simulink model "TRAMI_TM_CNT"  (R2018b)
settings: Solver=ode8  StartTime=0  StopTime=end_time  FixedStep=sampling_time  RelTol=1e-3
PreLoadFcn:
  | TRAMI_TM_CNT_PreLoad;
libraries: simulink x1
settings Model: Creator=nishimura  LastModifiedBy=E00026
settings DataIOCC: LimitDataPoints=on  SaveFormat=Array  SaveOutput=off  InspectSignalLogs=on  SaveTime=off
settings OptimizationCC: BlockReduction=off  BooleanDataType=off  LifeSpan=inf
settings DebuggingCC: SaveWithParameterizedLinksMsg=none  UnderspecifiedInitializationDetection=Classic  MergeDetectMultiDrivingBlocksExec=none  SignalResolutionControl=TryResolveAllWithWarning  ParameterPrecisionLossMsg=none  StrictBusMsg=ErrorOnBusTreatedAsVector  SFUnexpectedBacktrackingDiag=warning  SFNoUnconditionalDefaultTransitionDiag=warning  SFExecutionAtInitializationDiag=none
settings HardwareCC: ProdBitPerPointer=32  ProdBitPerSizeT=32  ProdBitPerPtrDiffT=32  ProdLargestAtomicFloat=None  ProdIntDivRoundTo=Undefined  ProdEndianess=Unspecified  ProdWordSize=32  ProdHWDeviceType=32-bit Generic  TargetUnknown=on
settings ModelReferenceCC: PropagateSignalLabelsOutOfModel=off
settings SFSimCC: SimUseLocalCustomCode=off
settings RTWCC: RTWUseLocalCustomCode=off
settings CodeAppCC: StateflowObjectComments=on
settings GRTTargetCC: TargetLangStandard=C89/C90 (ANSI)  GeneratePreprocessorConditionals=Disable all
settings ConfigComp: CovMetricSettings=dw  CovHtmlReporting=on  CovSaveCumulativeToWorkspaceVar=on  CovSaveSingleToWorkspaceVar=on  CovExternalEMLEnable=off  CovSFcnEnable=off

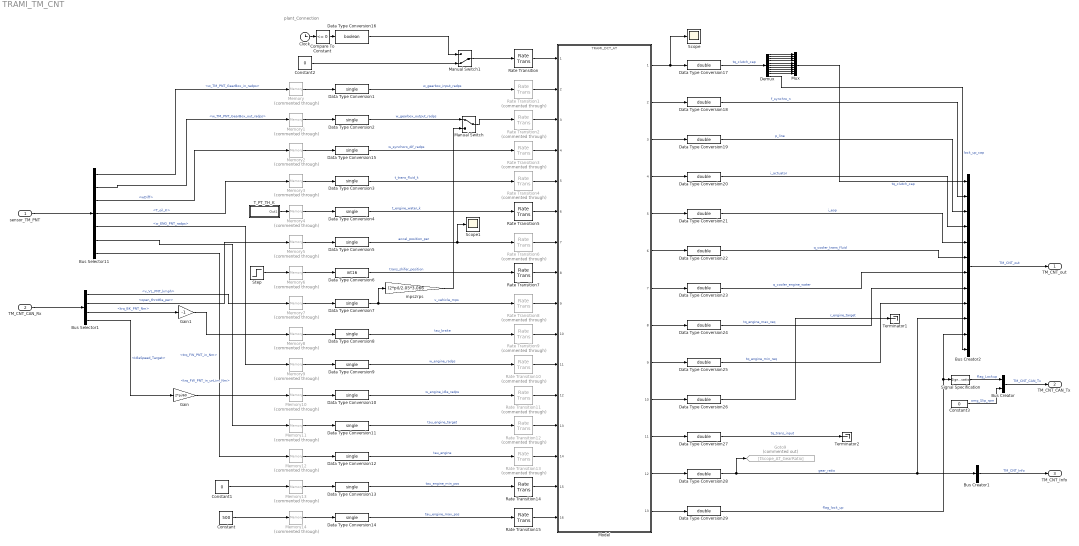
== system TRAMI_TM_CNT ==
  note: plant_Connection
  sensor_TM_PNT : Inport  OutDataTypeStr=Bus: sensor_TM_PNT_TRAMI  SampleTime=0.01
      settings: AttributesFormatString=|
      | <SampleTime = %<SampleTime>>
      | <%<OutDataTypeStr>>
  TM_CNT_CAN_Rx : Inport  Port=2  OutDataTypeStr=Bus: TM_CNT_CAN_Rx  SampleTime=0.01
      settings: AttributesFormatString=|
      | <SampleTime = %<SampleTime>>
      | <%<OutDataTypeStr>>
  Bus Creator : BusCreator  Inputs=2
  Bus Creator1 : BusCreator  Inputs=1
  Bus Creator2 : BusCreator  Inputs=12
  Bus Selector1 : BusSelector  OutputSignals=v_VL_PNT_kmph,open_throttle_per,trq_BK_PNT_Nm,IdleSpeed_Target
  Bus Selector11 : BusSelector  OutputSignals=w_TM_PNT_GearBox_in_radps,w_TM_PNT_GearBox_out_radps,wDiff,T_oil_K,w_ENG_PNT_radps,trq_FW_PNT_in_unLim_Nm,trq_FW_PNT_in_Nm
  Clock : Clock
  Compare To Constant : simulink/Logic and Bit Operations/Compare To Constant  relop=<=  const=0  OutDataTypeStr=boolean
  Constant : Constant  Value=500
  Constant1 : Constant  Value=0
  Constant2 : Constant  Value=0  OutDataTypeStr=boolean
  Constant3 : Constant  Value=0
  Data Type Conversion{1..5,7..15} (14 alike) : DataTypeConversion  OutDataTypeStr=single
  Data Type Conversion16 : DataTypeConversion  OutDataTypeStr=boolean
  Data Type Conversion{17..29} (13 alike) : DataTypeConversion  OutDataTypeStr=double
  Data Type Conversion6 : DataTypeConversion  OutDataTypeStr=int16
  Demux : Demux  Outputs=11
  Gain : Gain  Gain=2*pi/60
  Gain1 : Gain  Gain=-1
  Goto9 : Goto  Commented=on  GotoTag=tScope_AT_GearRatio
  Manual Switch : ManualSwitch
  Manual Switch1 : ManualSwitch  CurrentSetting=0
  Memory{,1..14} (15 alike) : Memory  Commented=through
  Model : ModelReference  ModelNameDialog=TRAMI_DCT_AT.slx  SimulationMode=Normal  ModelReferenceVersion=1.20
  Mux : Mux  Inputs=10
  Rate Transition{,5,7,14..15} (5 alike) : RateTransition
  Rate Transition{1..4,6,8..13} (11 alike) : RateTransition  Commented=through
  Scope : Scope
  Scope1 : Scope
  Signal Specification : SignalSpecification
  Step : Step  Time=5.57  SampleTime=0
  T_PT_TH_K : Subsystem
  Terminator1 : Terminator
  Terminator2 : Terminator
  mps2rps : Gain  Gain=(2*pi)/2.05*3.066
  TM_CNT_out : Outport  OutDataTypeStr=Bus: TM_CNT_TRAMI_out
      settings: AttributesFormatString=|
      | <SampleTime = %<SampleTime>>
      | <%<OutDataTypeStr>>
  TM_CNT_CAN_Tx : Outport  Port=2  OutDataTypeStr=Bus: TM_CNT_CAN_Tx
      settings: AttributesFormatString=|
      | <SampleTime = %<SampleTime>>
      | <%<OutDataTypeStr>>
  TM_CNT_Info : Outport  Port=3  OutDataTypeStr=Bus: TM_CNT_TRAMI_Info
      settings: AttributesFormatString=|
      | <SampleTime = %<SampleTime>>
      | <%<OutDataTypeStr>>
  wires:
  Bus Creator/1 -> TM_CNT_CAN_Tx/1  "TM_CNT_CAN_Tx"
  Bus Selector1/2 -> Memory5/1  "<open_throttle_per>"
  Bus Creator1/1 -> TM_CNT_Info/1  "TM_CNT_Info"
  Bus Selector11/6 -> Memory11/1  "<trq_FW_PNT_in_unLim_Nm>"
  Bus Selector11/3 -> Memory2/1  "<wDiff>"
  Bus Selector11/1 -> Memory/1  "<w_TM_PNT_GearBox_in_radps>"
  Bus Selector11/5 -> Memory9/1  "<w_ENG_PNT_radps>"
  Bus Selector11/2 -> Memory1/1  "<w_TM_PNT_GearBox_out_radps>"
  Bus Creator2/1 -> TM_CNT_out/1  "TM_CNT_out"
  sensor_TM_PNT/1 -> Bus Selector11/1
  Bus Selector11/4 -> Memory3/1  "<T_oil_K>"
  Bus Selector1/3 -> Gain1/1  "<trq_BK_PNT_Nm>"
  Bus Selector11/7 -> Memory12/1  "<trq_FW_PNT_in_Nm>"
  Bus Selector1/4 -> Gain/1  "<IdleSpeed_Target>"
  Bus Selector1/1 -> Memory7/1  "<v_VL_PNT_kmph>"
  TM_CNT_CAN_Rx/1 -> Bus Selector1/1
  Data Type Conversion29/1 -> Signal Specification/1, Bus Creator2/11  "flag_lock_up"
  Rate Transition15/1 -> Model/16
  Rate Transition14/1 -> Model/15
  Rate Transition13/1 -> Model/14
  Rate Transition12/1 -> Model/13
  Rate Transition11/1 -> Model/12
  Rate Transition10/1 -> Model/11
  Rate Transition9/1 -> Model/10
  Rate Transition8/1 -> Model/9
  Rate Transition7/1 -> Model/8
  Rate Transition6/1 -> Model/7
  Rate Transition5/1 -> Model/6
  Rate Transition4/1 -> Model/5
  Rate Transition3/1 -> Model/4
  Rate Transition2/1 -> Model/3
  Rate Transition1/1 -> Model/2
  Rate Transition/1 -> Model/1
  Demux/10 -> Mux/10
  Demux/9 -> Mux/9
  Demux/8 -> Mux/8
  Demux/7 -> Mux/7
  Demux/6 -> Mux/6
  Demux/5 -> Mux/5
  Demux/4 -> Mux/4
  Demux/3 -> Mux/3
  Demux/2 -> Mux/2
  Demux/1 -> Mux/1
  Demux/11 -> Bus Creator2/12  "lock_up_cap"
  Data Type Conversion17/1 -> Demux/1  "tq_clutch_cap"
  Data Type Conversion18/1 -> Bus Creator2/2  "f_synchro_n"
  Memory14/1 -> Data Type Conversion14/1
  Memory13/1 -> Data Type Conversion13/1
  Memory12/1 -> Data Type Conversion12/1
  Memory11/1 -> Data Type Conversion11/1
  Memory10/1 -> Data Type Conversion10/1
  Memory9/1 -> Data Type Conversion9/1
  Memory8/1 -> Data Type Conversion8/1
  Memory7/1 -> Data Type Conversion7/1
  Memory6/1 -> Data Type Conversion6/1
  Memory5/1 -> Data Type Conversion5/1
  Memory4/1 -> Data Type Conversion4/1
  Memory3/1 -> Data Type Conversion3/1
  Memory2/1 -> Data Type Conversion15/1
  Memory1/1 -> Data Type Conversion2/1
  Memory/1 -> Data Type Conversion1/1
  Data Type Conversion28/1 -> Goto9/1, Bus Creator1/1, Bus Creator2/10  "gear_ratio"
  Data Type Conversion27/1 -> Terminator2/1  "tq_trans_input"
  Data Type Conversion26/1 -> Terminator1/1  "r_engine_target"
  Data Type Conversion25/1 -> Bus Creator2/9  "tq_engine_min_req"
  Data Type Conversion24/1 -> Bus Creator2/8  "tq_engine_max_req"
  Data Type Conversion23/1 -> Bus Creator2/7  "q_cooler_engine_water"
  Data Type Conversion22/1 -> Bus Creator2/6  "q_cooler_trans_fluid"
  Data Type Conversion21/1 -> Bus Creator2/5  "i_eop"
  Data Type Conversion20/1 -> Bus Creator2/4  "i_actuator"
  Data Type Conversion19/1 -> Bus Creator2/3  "p_line"
  Mux/1 -> Bus Creator2/1  "tq_clutch_cap"
  Data Type Conversion7/1 -> mps2rps/1, Rate Transition8/1  "v_vehicle_mps"
  Data Type Conversion4/1 -> Rate Transition5/1  "t_engine_water_k"
  Data Type Conversion3/1 -> Rate Transition4/1  "t_trans_fluid_k"
  Data Type Conversion12/1 -> Rate Transition13/1  "tau_engine"
  Model/8 -> Data Type Conversion24/1
  Model/7 -> Data Type Conversion23/1
  Model/12 -> Data Type Conversion28/1
  Constant/1 -> Memory14/1
  Data Type Conversion10/1 -> Rate Transition11/1  "w_engine_idle_radps"
  T_PT_TH_K/1(Out1) -> Memory4/1
  Constant2/1 -> Manual Switch1/2
  Data Type Conversion6/1 -> Rate Transition7/1  "trans_shifer_position"
  Gain1/1 -> Memory8/1
  Data Type Conversion11/1 -> Rate Transition12/1  "tau_engine_target"
  Data Type Conversion14/1 -> Rate Transition15/1  "tau_engine_max_pos"
  Data Type Conversion13/1 -> Rate Transition14/1  "tau_engine_min_pos"
  Model/13 -> Data Type Conversion29/1
  Data Type Conversion15/1 -> Rate Transition3/1  "w_synchoro_dif_radps"
  Gain/1 -> Memory10/1
  Model/6 -> Data Type Conversion22/1
  Data Type Conversion9/1 -> Rate Transition10/1  "w_engine_radps"
  Data Type Conversion1/1 -> Rate Transition1/1  "w_gearbox_input_radps"
  Data Type Conversion2/1 -> Manual Switch/1  "w_gearbox_output_radps"
  Model/9 -> Data Type Conversion25/1
  Data Type Conversion5/1 -> Scope1/1, Rate Transition6/1  "accel_position_per"
  Step/1 -> Memory6/1
  Data Type Conversion8/1 -> Rate Transition9/1  "tau_brake"
  Model/5 -> Data Type Conversion21/1
  mps2rps/1 -> Manual Switch/2
  Model/11 -> Data Type Conversion27/1
  Model/1 -> Data Type Conversion17/1, Scope/1
  Model/3 -> Data Type Conversion19/1
  Model/4 -> Data Type Conversion20/1
  Model/2 -> Data Type Conversion18/1
  Constant1/1 -> Memory13/1
  Model/10 -> Data Type Conversion26/1
  Manual Switch/1 -> Rate Transition2/1
  Data Type Conversion16/1 -> Manual Switch1/1
  Clock/1 -> Compare To Constant/1
  Compare To Constant/1 -> Data Type Conversion16/1
  Manual Switch1/1 -> Rate Transition/1
  Signal Specification/1 -> Bus Creator/1  "flag_Lockup"
  Constant3/1 -> Bus Creator/2  "omg_Slip_rpm"

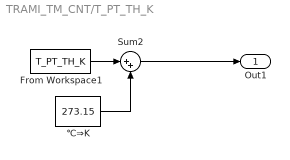
== system TRAMI_TM_CNT/T_PT_TH_K ==
  From Workspace1 : FromWorkspace  VariableName=T_PT_TH_K  SampleTime=0  OutputAfterFinalValue=Holding final value
  Sum2 : Sum  Inputs=|++
  ℃⇒K : Constant  Value=273.15
  Out1 : Outport
  wires:
  Sum2/1 -> Out1/1
  ℃⇒K/1 -> Sum2/2
  From Workspace1/1 -> Sum2/1
